simulink model "FIRP_NonLinear"  (R2021a)
settings: Solver=VariableStepAuto  StartTime=0.0  StopTime=10.0  RelTol=1e-3
values from neighbouring files (symbols this model uses):
  K = -(place(A,B,p))    [ass_7.m]
  L = Gamma - K*PI    [ass_7.m]
  w = 10    [ass_7.m]
settings Model: Creator=simon  LastModifiedBy=simon

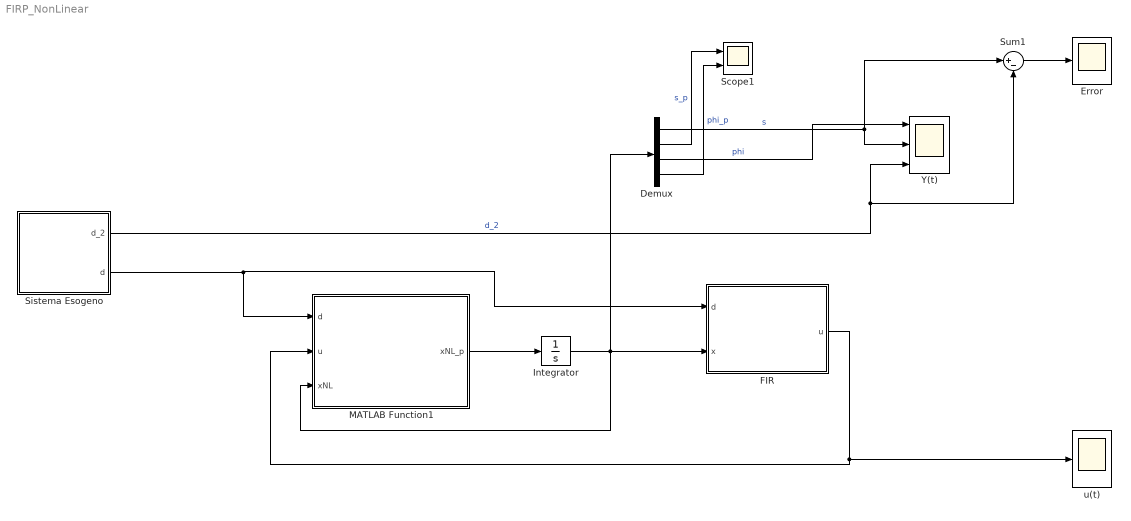
== system FIRP_NonLinear ==
  Demux : Demux
  Error : Scope
  FIR : Subsystem
  Integrator : Integrator
  MATLAB Function1 : MATLAB Function  TreatAsAtomicUnit=on
  Scope1 : Scope  NumInputPorts=2
  Sistema Esogeno : Subsystem
  Sum1 : Sum  Inputs=|+-
  Y(t) : Scope  NumInputPorts=3
  u(t) : Scope
  wires:
  FIR/1(u) -> MATLAB Function1/2(u), u(t)/1
  Demux/2 -> Scope1/1  "s_p"
  Demux/1 -> Y(t)/2, Sum1/1  "s"
  Integrator/1 -> MATLAB Function1/3(xNL), FIR/2(x), Demux/1
  Sum1/1 -> Error/1
  Demux/3 -> Y(t)/1  "phi"
  Sistema Esogeno/2(d) -> MATLAB Function1/1(d), FIR/1(d)
  Sistema Esogeno/1(d_2) -> Y(t)/3, Sum1/2  "d_2"
  MATLAB Function1/1(xNL_p) -> Integrator/1
  Demux/4 -> Scope1/2  "phi_p"

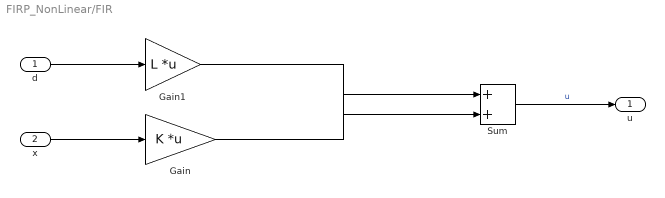
== system FIRP_NonLinear/FIR ==
  d : Inport
  x : Inport  Port=2
  Gain : Gain  Gain=K  Multiplication=Matrix(K*u)
  Gain1 : Gain  Gain=L  Multiplication=Matrix(K*u)
  Sum : Sum
  u : Outport
  wires:
  Gain1/1 -> Sum/2
  Sum/1 -> u/1  "u"
  Gain/1 -> Sum/1
  x/1 -> Gain/1
  d/1 -> Gain1/1

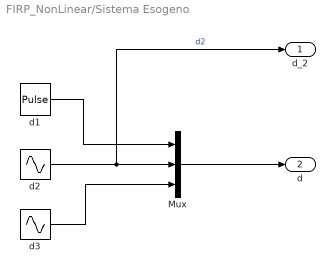
== system FIRP_NonLinear/Sistema Esogeno ==
  Mux : Mux  Inputs=3
  d1 : DiscretePulseGenerator  PulseType=Time based  Amplitude=0.5  Period=50  PulseWidth=50
  d2 : Sin  Frequency=w  SampleTime=0
  d3 : Sin  Frequency=w  Phase=pi/2  SampleTime=0
  d_2 : Outport
  d : Outport  Port=2
  wires:
  d3/1 -> Mux/3
  d2/1 -> d_2/1, Mux/2  "d2"
  d1/1 -> Mux/1
  Mux/1 -> d/1

== matlab function FIRP_NonLinear/MATLAB Function1 ==
  data: d input; u input; xNL_p output; xNL input
function xNL_p = NonLinearSpaceState(d,u,xNL)

M = 1;
l = 1;
F = 1;
g = 9.81;

xNL_p = zeros(4,1);

xNL_p(1)= xNL(2);
xNL_p(2)= (1/M)*(-F*xNL(2) + u + d(1));
xNL_p(3)= xNL(4);
xNL_p(4)= (g/l)*sin(xNL(3)) - (1/(M*l))*(-F*xNL(2) + u + d(1))*cos(xNL(3));
